simulink model "PC_Quadcopter_Simulation_Lyapnov_Hamilton_IAE"  (R2015b)
settings: Solver=FixedStepAuto  StartTime=0.0  StopTime=10  FixedStep=0.02  RelTol=1e-3
undefined symbols (not defined in the file): IC, quadModel
settings Model: Creator=HKJ  LastModifiedBy=HL

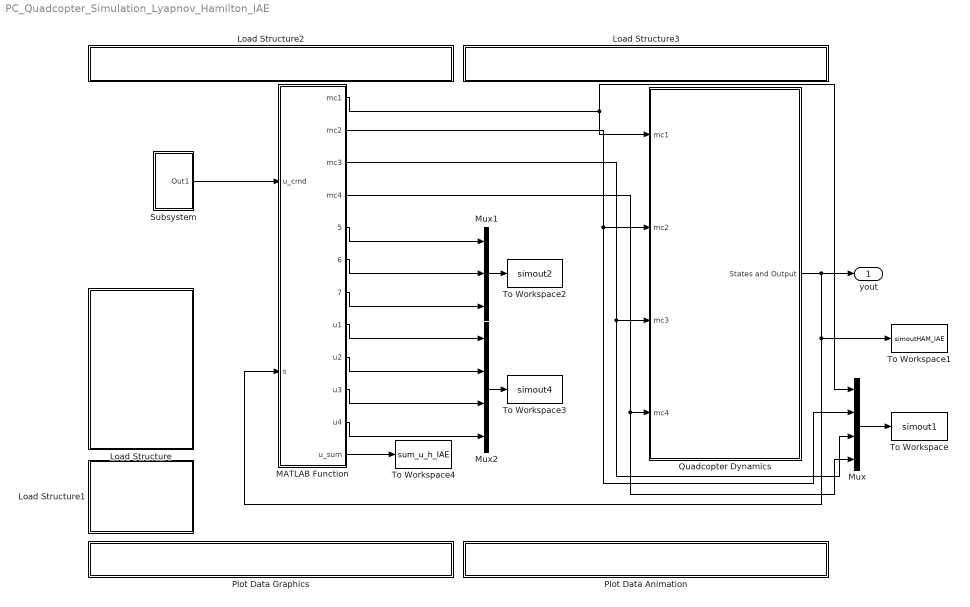
== system PC_Quadcopter_Simulation_Lyapnov_Hamilton_IAE ==
  Load Structure : Subsystem
      settings: OpenFcn=|
      | uiopen('load')
      | if (exist('IC')==1 && exist('quadModel')==1)
      | set_param(bdroot, 'SimulationCommand', 'update')
      | end
      mask Display: fprintf('LOAD:\nQuadcopter\nModel Or\nInitial\nConditions');
  Load Structure1 : Subsystem
      settings: OpenFcn=|
      | if (exist('IC')==1 && exist('quadModel')==1 && exist('yout') && exist('tout'))
      | saveSimResults()
      | else
      | msgbox('No Data To Save!')
      | end
      mask Display: fprintf('SAVE:\nSimulation\nResults');
  Load Structure2 : Subsystem
      settings: OpenFcn=|
      | if exist('GUI_Modeling') == 2,
      | run('GUI_Modeling')
      | 
      | else
      | 
      | msgbox('The desired GUI must be first added to MATLABs path.')
      | 
      | end
      mask Display: fprintf('OPEN GUI: Build New \n Model');
  Load Structure3 : Subsystem
      settings: OpenFcn=|
      | if exist('GUI_IC') == 2,
      | run('GUI_IC')
      | 
      | else
      | 
      | msgbox('The desired GUI must be first added to MATLABs path.')
      | 
      | end
      mask Display: fprintf('OPEN GUI: Create Initial \n Conditions');
  MATLAB Function : MATLAB Function  TreatAsAtomicUnit=on
  Mux : Mux
  Mux1 : Mux  Inputs=3
  Mux2 : Mux
  Plot Data Animation : Subsystem
      settings: OpenFcn=|
      | if exist('QuadAnim4') == 2,
      |     if exist('yout')
      | 	run('QuadAnim4');
      |     else
      |     msgbox('Simulation must be run before data can be plotted.');
      |     end
      | else                                                                          msgbox('The desired GUI must be first added to MATLABs path.')
      | end
      mask Display: fprintf('OPEN GUI: Flight Animation')
  Plot Data Graphics : Subsystem
      settings: OpenFcn=|
      | if exist('yout')
      | yout = evalin('base', 'yout');
      | tout = evalin('base', 'tout');
      | quadPlots(yout, tout)
      | else
      | msgbox('Simulation must be run before data can be plotted.')
      | end
      mask Display: fprintf('OPEN PLOT: State Data')
  Quadcopter Dynamics : Subsystem
  Subsystem : Subsystem
  To Workspace : ToWorkspace  VariableName=simout1  SampleTime=-1
      settings: Save2DSignal=2-D array (concatenate along first dimension)
  To Workspace1 : ToWorkspace  VariableName=simoutHAM_IAE  SampleTime=-1
      settings: Save2DSignal=2-D array (concatenate along first dimension)
  To Workspace2 : ToWorkspace  VariableName=simout2  SampleTime=-1
      settings: Save2DSignal=2-D array (concatenate along first dimension)
  To Workspace3 : ToWorkspace  VariableName=simout4  SampleTime=-1
      settings: Save2DSignal=2-D array (concatenate along first dimension)
  To Workspace4 : ToWorkspace  VariableName=sum_u_h_IAE  SampleTime=-1
      settings: Save2DSignal=2-D array (concatenate along first dimension)
  yout : Outport
  wires:
  Quadcopter Dynamics/1(States and Output) -> To Workspace1/1, MATLAB Function/2(s), yout/1
  MATLAB Function/1(mc1) -> Quadcopter Dynamics/1(mc1), Mux/1
  MATLAB Function/2(mc2) -> Quadcopter Dynamics/2(mc2), Mux/2
  MATLAB Function/3(mc3) -> Quadcopter Dynamics/3(mc3), Mux/3
  MATLAB Function/4(mc4) -> Quadcopter Dynamics/4(mc4), Mux/4
  Mux/1 -> To Workspace/1
  Subsystem/1(Out1) -> MATLAB Function/1(u_cmd)
  MATLAB Function/5(phi_cmd) -> Mux1/1
  MATLAB Function/6(the_cmd) -> Mux1/2
  MATLAB Function/7(psi_cmd) -> Mux1/3
  Mux1/1 -> To Workspace2/1
  MATLAB Function/9(u2) -> Mux2/2
  MATLAB Function/10(u3) -> Mux2/3
  MATLAB Function/11(u4) -> Mux2/4
  MATLAB Function/8(u1) -> Mux2/1
  Mux2/1 -> To Workspace3/1
  MATLAB Function/12(u_sum) -> To Workspace4/1

== system PC_Quadcopter_Simulation_Lyapnov_Hamilton_IAE/Load Structure ==

== system PC_Quadcopter_Simulation_Lyapnov_Hamilton_IAE/Load Structure1 ==

== system PC_Quadcopter_Simulation_Lyapnov_Hamilton_IAE/Load Structure2 ==

== system PC_Quadcopter_Simulation_Lyapnov_Hamilton_IAE/Load Structure3 ==

== system PC_Quadcopter_Simulation_Lyapnov_Hamilton_IAE/Plot Data Animation ==

== system PC_Quadcopter_Simulation_Lyapnov_Hamilton_IAE/Plot Data Graphics ==

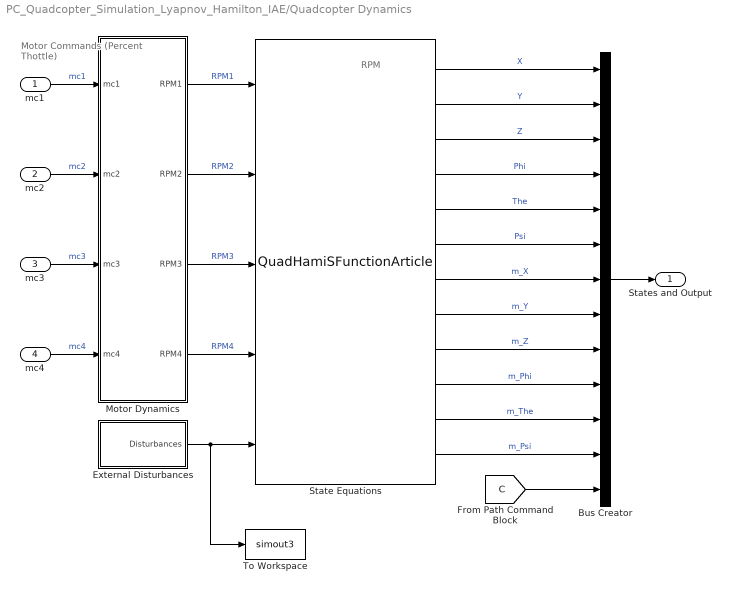
== system PC_Quadcopter_Simulation_Lyapnov_Hamilton_IAE/Quadcopter Dynamics ==
  note: Motor Commands
      | (Percent Thottle)
  note: RPM
  mc1 : Inport
  mc2 : Inport  Port=2
  mc3 : Inport  Port=3
  mc4 : Inport  Port=4
  Bus Creator : BusCreator  Inputs='X','Y','Z','Phi','The','Psi','m_X','m_Y','m_Z','m_Phi','m_The','m_Psi','XY_Cmd'
  External Disturbances : Subsystem
  Motor Dynamics : Subsystem
  State Equations : M-S-Function  FunctionName=QuadHamiSFunctionArticle  Parameters=quadModel,IC
      mask Display:
      | port_label('input', 1, 'RPM1')
      | port_label('input', 2, 'RPM2')
      | port_label('input', 3, 'RPM3')
      | port_label('input', 4, 'RPM4')
      | port_label('input', 5, 'Disturbances')
      | port_label('output', 1, 'X')
      | port_label('output', 2, 'Y')
      | port_label('output', 3, 'Z')
      | port_label('output', 4, 'Phi')
      | port_label('output', 5, 'The')
      | port_label('output', 6, 'Psi')
      | port_label('output', 7, 'm_X')
      | port_label('output', 8, 'm_Y')
      | port_label('output', 9, 'm_Z')
      | port_label('output', 10, 'm_Phi')
      | port_label('output', 11, 'm_The')
      | port_label('output', 12, 'm_Psi')
  To Workspace : ToWorkspace  VariableName=simout3  SampleTime=-1
      settings: Save2DSignal=2-D array (concatenate along first dimension)
  States and Output : Outport
  wires:
  mc1/1 -> Motor Dynamics/1(mc1)  "mc1"
  mc2/1 -> Motor Dynamics/2(mc2)  "mc2"
  mc3/1 -> Motor Dynamics/3(mc3)  "mc3"
  mc4/1 -> Motor Dynamics/4(mc4)  "mc4"
  State Equations/1 -> Bus Creator/1  "X"
  State Equations/2 -> Bus Creator/2  "Y"
  State Equations/3 -> Bus Creator/3  "Z"
  State Equations/4 -> Bus Creator/4  "Phi"
  State Equations/5 -> Bus Creator/5  "The"
  State Equations/6 -> Bus Creator/6  "Psi"
  State Equations/7 -> Bus Creator/7  "m_X"
  State Equations/8 -> Bus Creator/8  "m_Y"
  State Equations/9 -> Bus Creator/9  "m_Z"
  State Equations/10 -> Bus Creator/10  "m_Phi"
  State Equations/11 -> Bus Creator/11  "m_The"
  State Equations/12 -> Bus Creator/12  "m_Psi"
  Bus Creator/1 -> States and Output/1
  Motor Dynamics/1(RPM1) -> State Equations/1  "RPM1"
  Motor Dynamics/2(RPM2) -> State Equations/2  "RPM2"
  Motor Dynamics/3(RPM3) -> State Equations/3  "RPM3"
  Motor Dynamics/4(RPM4) -> State Equations/4  "RPM4"
  External Disturbances/1("Disturbances ") -> To Workspace/1, State Equations/5
  [C] -> Bus Creator/13

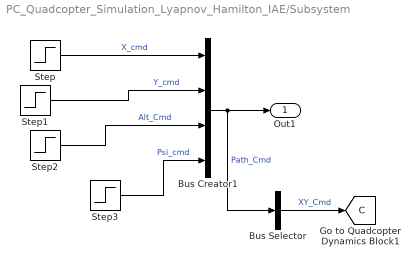
== system PC_Quadcopter_Simulation_Lyapnov_Hamilton_IAE/Subsystem ==
  Bus Creator1 : BusCreator  Inputs=4
  Bus Selector : BusSelector  OutputSignals=X_cmd,Y_cmd  OutputAsBus=on
  Step : Step  Time=0
  Step1 : Step  Time=0
  Step2 : Step  Time=0  After=-1
  Step3 : Step  Time=0  After=0
  Out1 : Outport
  tag scope: C=global
  wires:
  Step3/1 -> Bus Creator1/4  "Psi_cmd"
  Step2/1 -> Bus Creator1/3  "Alt_Cmd"
  Step/1 -> Bus Creator1/1  "X_cmd"
  Step1/1 -> Bus Creator1/2  "Y_cmd"
  Bus Creator1/1 -> Bus Selector/1, Out1/1  "Path_Cmd"
  Bus Selector/1 -> [C]  "XY_Cmd"

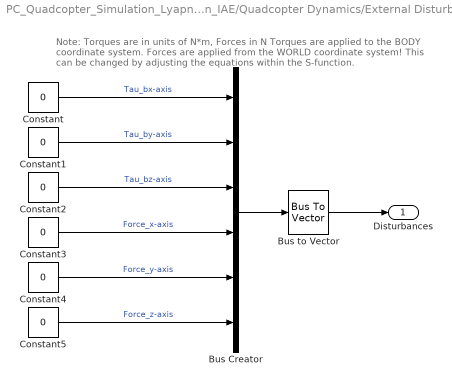
== system PC_Quadcopter_Simulation_Lyapnov_Hamilton_IAE/Quadcopter Dynamics/External Disturbances ==
  note: Note: Torques are in units of N*m, Forces in N
      | Torques are applied to the BODY coordinate system.
      | Forces are applied from the WORLD coordinate system!
      | This can be changed by adjusting the equations within the S-function.
  Bus Creator : BusCreator  Inputs=6
  Bus to Vector : BusToVector
  Constant{,1..5} (6 alike) : Constant  Value=0
  "Disturbances " : Outport
  wires:
  Bus to Vector/1 -> "Disturbances "/1
  Bus Creator/1 -> Bus to Vector/1
  Constant/1 -> Bus Creator/1  "Tau_bx-axis"
  Constant1/1 -> Bus Creator/2  "Tau_by-axis"
  Constant2/1 -> Bus Creator/3  "Tau_bz-axis"
  Constant3/1 -> Bus Creator/4  "Force_x-axis"
  Constant4/1 -> Bus Creator/5  "Force_y-axis"
  Constant5/1 -> Bus Creator/6  "Force_z-axis"

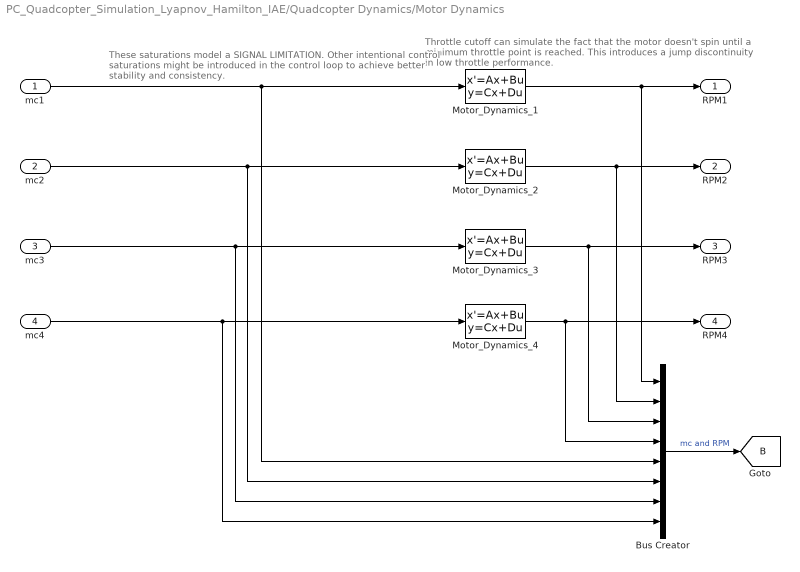
== system PC_Quadcopter_Simulation_Lyapnov_Hamilton_IAE/Quadcopter Dynamics/Motor Dynamics ==
  note: Throttle cutoff can simulate the fact that the motor doesn't
      | spin until a minimum throttle point is reached. This introduces
      | a jump discontinuity in low throttle performance.
  note: These saturations model a SIGNAL LIMITATION.
      | Other intentional control saturations might be introduced in the
      | control loop to achieve better stability and consistency.
  mc1 : Inport
  mc2 : Inport  Port=2
  mc3 : Inport  Port=3
  mc4 : Inport  Port=4
  Bus Creator : BusCreator  Inputs=8
  Motor_Dynamics_1 : StateSpace  A=-1/quadModel.T  C=1/quadModel.T  D=0  X0=IC.w1*quadModel.T
  Motor_Dynamics_2 : StateSpace  A=-1/quadModel.T  C=1/quadModel.T  D=0  X0=IC.w2*quadModel.T
  Motor_Dynamics_3 : StateSpace  A=-1/quadModel.T  C=1/quadModel.T  D=0  X0=IC.w3*quadModel.T
  Motor_Dynamics_4 : StateSpace  A=-1/quadModel.T  C=1/quadModel.T  D=0  X0=IC.w4*quadModel.T
  RPM1 : Outport
  RPM2 : Outport  Port=2
  RPM3 : Outport  Port=3
  RPM4 : Outport  Port=4
  tag scope: B=global
  wires:
  mc1/1 -> Motor_Dynamics_1/1, Bus Creator/5
  mc2/1 -> Motor_Dynamics_2/1, Bus Creator/6
  mc3/1 -> Motor_Dynamics_3/1, Bus Creator/7
  mc4/1 -> Motor_Dynamics_4/1, Bus Creator/8
  Motor_Dynamics_1/1 -> Bus Creator/1, RPM1/1
  Motor_Dynamics_2/1 -> Bus Creator/2, RPM2/1
  Motor_Dynamics_3/1 -> Bus Creator/3, RPM3/1
  Motor_Dynamics_4/1 -> Bus Creator/4, RPM4/1
  Bus Creator/1 -> [B]  "mc and RPM"

== matlab function PC_Quadcopter_Simulation_Lyapnov_Hamilton_IAE/MATLAB Function ==
  data: u_cmd input; mc1 output; s input; mc2 output; mc3 output; mc4 output; phi_cmd output; the_cmd output; psi_cmd output; u1 output; u2 output; u3 output; u4 output; u_sum output
function [mc1,mc2,mc3,mc4,phi_cmd,the_cmd,psi_cmd, u1,u2,u3,u4, u_sum] = fcn(u_cmd,s)
%自己设计的控制器
k1 = 4.1649;
k2 = 8;
k3 = 4.1649;
k4 = 8;
k5 = 2.0291;
k6 = 2.5;
k7= 0.9548;
k8= 2.5671;
k9 = 0.9548;
k10 = 2.5671;
k11 = 1.7491;
k12 = 4.9313;
Ix = 0.0094999;Iy=0.0094999;Iz=0.018576;
I = [Ix,0,0;0,Iy,0;0,0,Iz];
m=1.023;g=9.81;
% L=0.185738;%z这个值有问题
ct=1.4865e-07;
cq=2.925e-09;
ctl = 3.30374625e-08;

x_cmd = u_cmd(1);
y_cmd = u_cmd(2);
alt_cmd = u_cmd(3);
psi_cmd = u_cmd(4);
x = s(1);y = s(2);z = s(3);
Phi = s(4);The = s(5);Psi = s(6);
m_x = s(7);m_y = s(8);m_z = s(9);
m_Phi = s(10);m_The = s(11);m_Psi = s(12);

dPhi = (Iy*Iz+(Ix-Iz)*Iy*sin(The)^2-(Iy-Iz)*Ix*sin(Phi)^2*sin(The)^2)*m_Phi/(Ix*Iy*Iz*cos(The)^2)+...
       (-(Iy-Iz)*cos(Phi)*sin(Phi)*sin(The)*m_The)/(Iy*Iz*cos(The))+...
       (Iy*cos(Phi)^2+Iz*sin(Phi)^2)*sin(The)*m_Psi/(Iy*Iz*cos(The)^2);
dThe = -(Iy-Iz)*cos(Phi)*sin(Phi)*sin(The)*m_Phi/(Iy*Iz*cos(The))+...
       (Iy*sin(Phi)^2+Iz*cos(Phi)^2)*m_The/(Iy*Iz)+...
       (-(Iy-Iz)*cos(Phi)*sin(Phi))*m_Psi/(Iy*Iz*cos(The));
dPsi = (Iy*cos(Phi)^2+Iz*sin(Phi)^2)*sin(The)*m_Phi/(Iy*Iz*cos(The)^2)+...
       (-(Iy-Iz)*cos(Phi)*sin(Phi))*m_The/(Iy*Iz*cos(The))+...
       (Iy*cos(Phi)^2+Iz*sin(Phi)^2)*m_Psi/(Iy*Iz*cos(The)^2);

g1 = (Iy*Iz+(Ix-Iz)*Iy*sin(The)^2-(Iy-Iz)*Ix*sin(Phi)^2*sin(The)^2)/(Ix*Iy*Iz*cos(The)^2);
g2 = (Iy*sin(Phi)^2+Iz*cos(Phi)^2)/(Iy*Iz);
g3 = (Iy*cos(Phi)^2+Iz*sin(Phi)^2)/(Iy*Iz*cos(The)^2);

g12 = -(Iy-Iz)*cos(Phi)*sin(Phi)*sin(The)/(Iy*Iz*cos(The));
g13 = (Iy*cos(Phi)^2+Iz*sin(Phi)^2)*sin(The)/(Iy*Iz*cos(The)^2);
g23 = -(Iy-Iz)*cos(Phi)*sin(Phi)/(Iy*Iz*cos(The));

J = [g1,g12,g13;g12,g2,g23;g13,g23,g3];

f1 = -(Iy-Iz)*(dThe^2*sin(Phi)*cos(Phi)-dThe*dPsi*cos(2*Phi)*cos(The)-dPsi^2*sin(Phi)*cos(Phi)*cos(The)^2);
f2 = (Ix-Iy*sin(Phi)^2-Iz*cos(Phi)^2)*dPsi^2*sin(The)*cos(The)-(Iy-Iz)*dThe*dPsi*sin(Phi)*cos(Phi)*sin(The)-dPhi*dPsi*Ix*cos(The);


e7 = x - x_cmd;
e8 = m_x/m + k7*e7;
e9 = y - y_cmd;
e10 = m_y/m + k9*e9;
e11 = z-alt_cmd;
e12 = m_z/m+k11*e11;

alpha1 = m*((k7^2-1)*e7-(k7+k8)*e8);
alpha2 = m*((k9^2-1)*e9-(k9+k10)*e10);
alpha3 = -m*g+m*((k11^2-1)*e11-(k11+k12)*e12);
beta1 = alpha1*cos(Psi) + alpha2*sin(Psi);
beta2 = -alpha1*sin(Psi) + alpha2*cos(Psi);
beta3 = alpha3;
the_cmd = atan(beta1/beta3);
phi_cmd = atan(-beta2*cos(the_cmd)/beta3);
u1 = beta3/(cos(phi_cmd)*cos(the_cmd));

e1 = Phi-phi_cmd;
e2 = m_Phi/Ix+k1*e1;
e3 = The-the_cmd;
e4 = m_The/Iy+k3*e3;
e5 = Psi-psi_cmd;
e6 = m_Psi/Iz+k5*e5;

K_eta = [k1,0,0;0,k3,0;0,0,k5];
K_peta = [k2,0,0;0,k4,0;0,0,k6];
e_eta = [e1;e3;e5];
e_peta = [e2;e4;e6];
tau_p=I*((K_eta*J*I*K_eta-J*I)*e_eta-(K_eta+K_peta)*J*I*e_peta)-[f1;f2;0];
u2 = tau_p(1);
u3 = tau_p(2);
u4 = tau_p(3);

% 
% u2 = -f1+(-(k1*g1*Ix+k2)*e2+(g1*Ix*k1^2-g1*Ix)*e1)*Ix;
% u3 = -f2+(-(k3*g2*Iy+k4)*e4+(g2*Iy*k3^2-g2*Iy)*e3)*Iy;
% u4 =(-(k5*g3*Iz+k6)*e6+(g3*Iz*k5^2-g3*Iz)*e5)*Iz;

mc1 = sqrt((-u1/ct+u4/cq)*0.25+u3/ctl*0.5);
mc2 = sqrt((-u1/ct-u4/cq)*0.25+u2/ctl*0.5);
mc3 = sqrt((-u1/ct+u4/cq)*0.25-u3/ctl*0.5);
mc4 = sqrt((-u1/ct-u4/cq)*0.25-u2/ctl*0.5);

u_sum = u1*u1+u2*u2+u3*u3+u4*u4;
